simulink model "Q5_30"  (R2015b)
settings: Solver=VariableStepAuto  StartTime=0.0  StopTime=10000  RelTol=1e-3
settings Model: Creator=sjt85  LastModifiedBy=sjt85

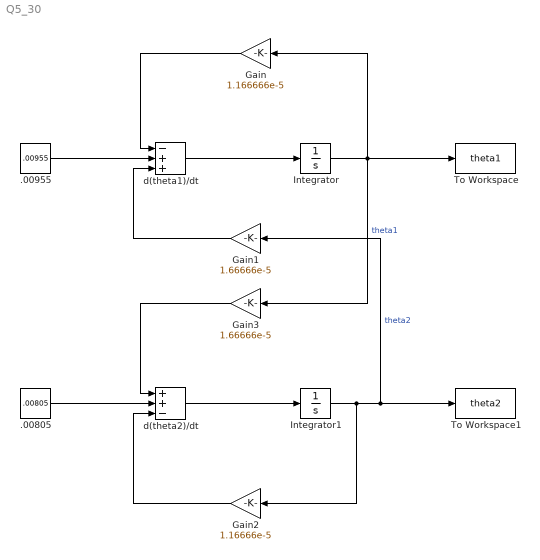
== system Q5_30 ==
  .00805 : Constant  Value=.00805
  .00955 : Constant  Value=.00955
  Gain : Gain  Gain=1.166666e-5
  Gain1 : Gain  Gain=1.66666e-5
  Gain2 : Gain  Gain=1.16666e-5
  Gain3 : Gain  Gain=1.66666e-5
  Integrator : Integrator  InitialCondition=20
  Integrator1 : Integrator  InitialCondition=20
  To Workspace : ToWorkspace  VariableName=theta1  SaveFormat=Timeseries  SampleTime=-1
  To Workspace1 : ToWorkspace  VariableName=theta2  SaveFormat=Timeseries  SampleTime=-1
  d(theta1)/dt : Sum  Inputs=-|+|+
  d(theta2)/dt : Sum  Inputs=+|+|-
  wires:
  d(theta1)/dt/1 -> Integrator/1
  Integrator/1 -> Gain3/1, Gain/1, To Workspace/1  "theta1"
  d(theta2)/dt/1 -> Integrator1/1
  Integrator1/1 -> Gain2/1, Gain1/1, To Workspace1/1  "theta2"
  Gain/1 -> d(theta1)/dt/1
  Gain1/1 -> d(theta1)/dt/3
  .00955/1 -> d(theta1)/dt/2
  .00805/1 -> d(theta2)/dt/2
  Gain2/1 -> d(theta2)/dt/3
  Gain3/1 -> d(theta2)/dt/1
